simulink model "ex3_sim1"  (R2018b)
settings: Solver=ode45  StartTime=0.0  StopTime=0.5  MaxStep=0.001  RelTol=1e-3  EnableMultiTasking=on
undefined symbols (not defined in the file): Ar, degs2rpm, denCd, denHd, km, numCd, numHd, rpm2rads, t0r, Tm, Ts
settings Model: Creator=antonello  LastModifiedBy=riccardo
settings DataIOCC: LimitDataPoints=on  SaveFormat=Array
settings OptimizationCC: LifeSpan=inf
settings DebuggingCC: SolverPrmCheckMsg=warning  LibraryContextMissingDiagnostic=none  SFUnexpectedBacktrackingDiag=warning  SFNoUnconditionalDefaultTransitionDiag=warning  SFExecutionAtInitializationDiag=none
settings HardwareCC: ProdBitPerPointer=32  ProdBitPerSizeT=32  ProdBitPerPtrDiffT=32  ProdLargestAtomicFloat=None  ProdIntDivRoundTo=Undefined  ProdEndianess=Unspecified  ProdWordSize=32  ProdHWDeviceType=32-bit Generic
settings ModelReferenceCC: PropagateSignalLabelsOutOfModel=off
settings SFSimCC: SimUseLocalCustomCode=off
settings RTWCC: RTWUseLocalCustomCode=off
settings CodeAppCC: StateflowObjectComments=on
settings GRTTargetCC: TargetLangStandard=C89/C90 (ANSI)  GeneratePreprocessorConditionals=Disable all
settings ConfigComp: CovMetricSettings=dw  CovHtmlReporting=on  CovSaveCumulativeToWorkspaceVar=on  CovSaveSingleToWorkspaceVar=on  CovExternalEMLEnable=off  CovSFcnEnable=off

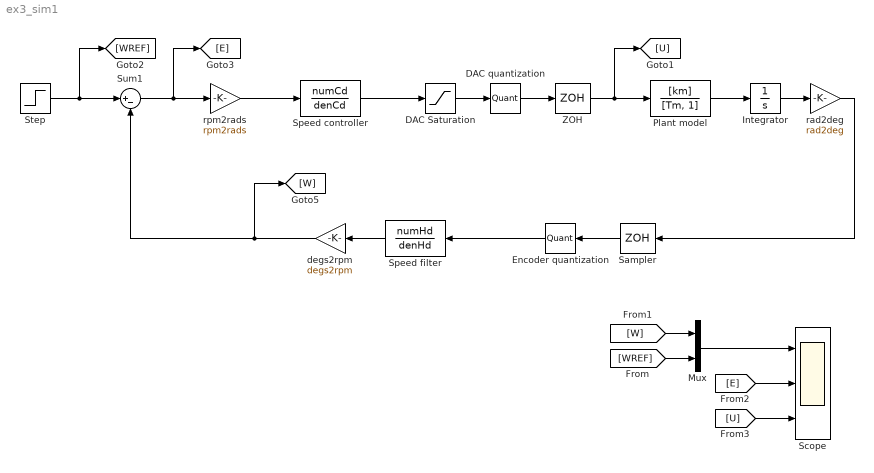
== system ex3_sim1 ==
  DAC Saturation : Saturate  UpperLimit=10  LowerLimit=-10
  DAC quantization : Quantizer  QuantizationInterval=qdac
  Encoder quantization : Quantizer  QuantizationInterval=qenc
  Integrator : Integrator
  Mux : Mux  Inputs=2
  Plant model : TransferFcn  Numerator=[km]  Denominator=[Tm, 1]
  Sampler : ZeroOrderHold  SampleTime=Ts
  Scope : Scope  NumInputPorts=3
  Speed controller : DiscreteTransferFcn  Numerator=numCd  Denominator=denCd  SampleTime=Ts
  Speed filter : DiscreteTransferFcn  Numerator=numHd  Denominator=denHd
  Step : Step  Time=t0r  After=Ar  SampleTime=0
  Sum1 : Sum  Inputs=|+-
  ZOH : ZeroOrderHold  SampleTime=Ts
  degs2rpm : Gain  Gain=degs2rpm
  rad2deg : Gain  Gain=rad2deg
  rpm2rads : Gain  Gain=rpm2rads
  wires:
  Sum1/1 -> [E], rpm2rads/1
  Step/1 -> [WREF], Sum1/1
  [W] -> Mux/1
  [WREF] -> Mux/2
  rpm2rads/1 -> Speed controller/1
  DAC Saturation/1 -> DAC quantization/1
  Mux/1 -> Scope/1
  [E] -> Scope/2
  [U] -> Scope/3
  ZOH/1 -> Plant model/1, [U]
  Speed filter/1 -> degs2rpm/1
  degs2rpm/1 -> Sum1/2, [W]
  Plant model/1 -> Integrator/1
  Integrator/1 -> rad2deg/1
  rad2deg/1 -> Sampler/1
  Speed controller/1 -> DAC Saturation/1
  DAC quantization/1 -> ZOH/1
  Sampler/1 -> Encoder quantization/1
  Encoder quantization/1 -> Speed filter/1
